simulink model "pmsm_ctrl"  (R2018a)
settings: Solver=FixedStepDiscrete  StartTime=0.0  StopTime=3  FixedStep=FastTsample / 10.  RelTol=1e-3  EnableMultiTasking=on
model workspace (MATLAB code in the model file):
  | cmdLim = Simulink.Parameter;
  | cmdLim.Value = 15;
  | cmdLim.Description = 'Limit for controlling the maximum surface command angle.';
  | cmdLim.Min = 0;
  | cmdLim.Max = 90;
  | cmdLim.DocUnits = 'deg';
  | 
  | dispGain = Simulink.Parameter;
  | dispGain.Value = 0.75;
  | dispGain.Description = 'Gain applied to the displacement error.';
  | dispGain.Min = 0;
  | dispGain.Max = [];
  | dispGain.DocUnits = 'deg/sec/deg';
  | 
  | dispLim = Simulink.Parameter;
  | dispLim.Value = 30;
  | dispLim.Description = 'Limit for controlling the maximum commanded angle.';
  | dispLim.Min = 0;
  | dispLim.Max = 180;
  | dispLim.DocUnits = 'deg';
  | 
  | intGain = Simulink.Parameter;
  | intGain.Value = 0.5;
  | intGain.Description = 'Gain applied to the integral error.';
  | intGain.Min = 0;
  | intGain.Max = [];
  | intGain.DocUnits = 'deg/sec/deg/sec';
  | 
  | intLim = Simulink.Parameter;
  | intLim.Value = 5;
  | intLim.Description = 'Limit for controlling the maximum commanded angle.';
  | intLim.Min = 0;
  | intLim.Max = 90;
  | intLim.DocUnits = 'deg';
  | 
  | rateGain = Simulink.Parameter;
  | rateGain.Value = 2;
  | rateGain.Description = 'Gain applied to the rate error.';
  | rateGain.Min = 0;
  | rateGain.Max = [];
  | rateGain.DocUnits = 'deg/deg/sec';
  | 
  | rateLim = Simulink.Parameter;
  | rateLim.Value = 6;
  | rateLim.Description = 'Limit for controlling the maximum commanded angle.';
  | rateLim.Min = 0;
  | rateLim.Max = 180;
  | rateLim.DocUnits = 'deg/sec';
  | 
  | hdgGain = Simulink.Parameter;
  | hdgGain.Value = 0.015;
undefined symbols (not defined in the file): CalMgrSt_T, Cfg_AutoCalEnbl, Cfg_EnblDynComp, Cfg_EncCnts, Cfg_IfbkCtrlBW, Cfg_MtrJm, Cfg_MtrKf, Cfg_MtrKtrq, Cfg_SpdCtrlBW, Cfg_SpdSnsEnbl, Cfg_StepToEncCnts, Cfg_UseObsPosEst, DiscIntNeverNeededParam, DistObs_J, DistObs_K1, DistObs_K2, DistObs_K3, EncCntsToRads, MtrCtrlCal_T, MtrCtrlMd, MtrCtrlMd_T, MtrParams, TsFast, TsMain
libraries: ctrl_lib x15, simulink x10, peTransforms x1, adrc_lib x1
(part 2 of 2)

== stateflow chart pmsm_ctrl/CalibRoutines/mtr_ifbk_ofs_ident/ResIdCal ==
  state mtr_angl_ofs_cal_actv
    en, du:
    CtrlMdRqst = MtrCtrlMd_T.CTRL_MD_RAW_PWM;
    PwmRqst = 0.0;
    CalMgrStRqst = CalMgrSt_T.ST_IFBK_OFS_CAL;
    ifbk_abc_sum = get_mtr_ifbk_sum(MtrIfbk);
    CalData_IfbkOfs_Abc[0] = 0.;
    CalData_IfbkOfs_Abc[1] = 0.;
    CalData_IfbkOfs_Abc[2] = 0.;
  state mtr_ifbk_sum_abc = get_mtr_ifbk_sum(mtr_ifbk_abc) [function]
  state mtr_ifbk_avg_abc = get_mtr_ifbk_avg(mtr_ifbk_sum_abc, ncycles) [function]
  state mtr_angl_ofs_cal_done
    en, du:
    CtrlMdRqst = MtrCtrlMd_T.CTRL_MD_OFF;
    CalMgrStRqst = CalMgrSt_T.ST_DONE;
    PwmRqst = 0.0;
    CalData_IfbkOfs_Abc = get_mtr_ifbk_avg(ifbk_abc_sum, TICK_WAIT_SETTLE);
  (default) -> mtr_angl_ofs_cal_actv
  mtr_angl_ofs_cal_actv -> mtr_angl_ofs_cal_done : [after(TICK_WAIT_SETTLE, tick)] // Wait for motor to settle.
  data: mtr_ifbk_abc function_input size=3; mtr_ifbk_sum_abc function_output; mtr_ifbk_sum_abc function_input size=3; mtr_ifbk_avg_abc function_output; ncycles function_input; CtrlMdRqst output; CalMgrStRqst output; PwmRqst output single; ifbk_abc_sum local single size=3; MtrIfbk input size=3; CalData_IfbkOfs_Abc data_store_memory; TICK_WAIT_SETTLE constant uint32 =100

== stateflow chart pmsm_ctrl/CalibRoutines/enc_ofs_cal_routine/EncOfsCal ==
  state mtr_n_poles_enc_ofs_init
    en, du:
    CtrlMdRqst = MtrCtrlMd_T.CTRL_MD_RAW_PWM;
    PwmRqst = Cfg_AnglOfsCalPwmDuty;
    CalMgrStRqst = CalMgrSt_T.ST_ENC_OFS;
    CalData_EncOfs = 0;
    CalData_nPoles = -1;
    Ticks = 0;
    ticks_inc = int32(TICKS_TGT / TICKS_OFS_CAL_RAMP);
    ticks_start = 0;
    ticks_end = 0;
  state calc_enc_ofs_move_forward
    en:
    ticks_start = EncCnts;
    CalData_EncOfs = ticks_start;
    en, du:
    Ticks += ticks_inc;
  state calc_n_poles
    en:
    ticks_end = EncCnts;
    en, du:
    Ticks = Ticks;
    CalData_nPoles = int32(Ticks / (ticks_end - ticks_start))
  state move_back_calc_enc_ofs
    en, du:
    Ticks -= ticks_inc;
  state done
    en, du:
    CtrlMdRqst = MtrCtrlMd_T.CTRL_MD_OFF;
    CalMgrStRqst = CalMgrSt_T.ST_DONE;
    PwmRqst = 0.;
  (default) -> mtr_n_poles_enc_ofs_init
  mtr_n_poles_enc_ofs_init -> calc_enc_ofs_move_forward : [after(WAIT_SETTLE_TICKS, tick)] // Wait for motor / current to settle.
  calc_enc_ofs_move_forward -> calc_n_poles : [Ticks >= TICKS_TGT]
  calc_n_poles -> move_back_calc_enc_ofs : [after(WAIT_SETTLE_TICKS, tick)]
  move_back_calc_enc_ofs -> done : [Ticks <= 0]
  data: Cfg_AnglOfsCalPwmDuty parameter size=1; EncCnts input size=1; CtrlMdRqst output; CalMgrStRqst output; PwmRqst output single; CalData_EncOfs data_store_memory; Ticks output int32; ticks_inc local int32; ticks_tgt local int32; CalData_nPoles data_store_memory; ticks_start local int32; ticks_end local int32; TICKS_TGT constant int32 =8 * Cfg_EncCnts; WAIT_SETTLE_TICKS constant uint32 =100; TICKS_OFS_CAL_RAMP constant uint32 =500

== stateflow chart pmsm_ctrl/CalibRoutines/mtr_res_ident/ResIdCal ==
  state res_id_init
    en, du:
    CtrlMdRqst = MtrCtrlMd_T.CTRL_MD_RAW_PWM;
    PwmRqst = PWM_R_CAL_DUTY;
    CalMgrStRqst = CalMgrSt_T.ST_RES_ID;
    ifbk_sum = 0;
    CalData_Res = -1.0;
  state res_id_actv
    en, du:
    ifbk_sum += MtrIfbk;
  state done
    en, du:
    CtrlMdRqst = MtrCtrlMd_T.CTRL_MD_OFF;
    CalMgrStRqst = CalMgrSt_T.ST_DONE;
    PwmRqst = 0.;
    CalData_Res = PWM_R_CAL_DUTY * (2. / 3.) * (MtrParams.Vdc / 2.) / (ifbk_sum / TICK_R_CAL);
  (default) -> res_id_init
  res_id_init -> res_id_actv : [after(TICK_WAIT_SETTLE, tick)] // Wait for current / motor to settle.
  res_id_actv -> done : [after(TICK_R_CAL, tick)]
  data: CtrlMdRqst output; CalMgrStRqst output; PwmRqst output single; ifbk_sum local single =0.; MtrIfbk input; CalData_Res data_store_memory; MtrParams parameter; PWM_R_CAL_DUTY constant single =0.05; CAL_I_TGT constant single =1.5; TICK_WAIT_SETTLE constant uint32 =30; TICK_R_CAL constant uint32 =100
